simulink model "FMC_TopLevel_Model"  (R2025a)
settings: Solver=VariableStepAuto  StartTime=0.0  StopTime=10.0  RelTol=1e-3
settings Model: Creator=mu22504  LastModifiedBy=Adam

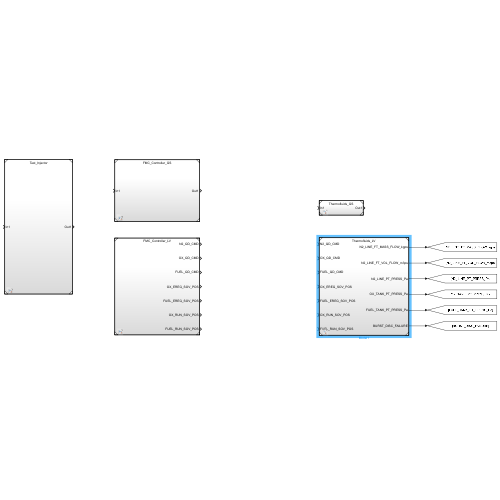
[thumbnail: Simulink's stored preview of the top-level diagram]
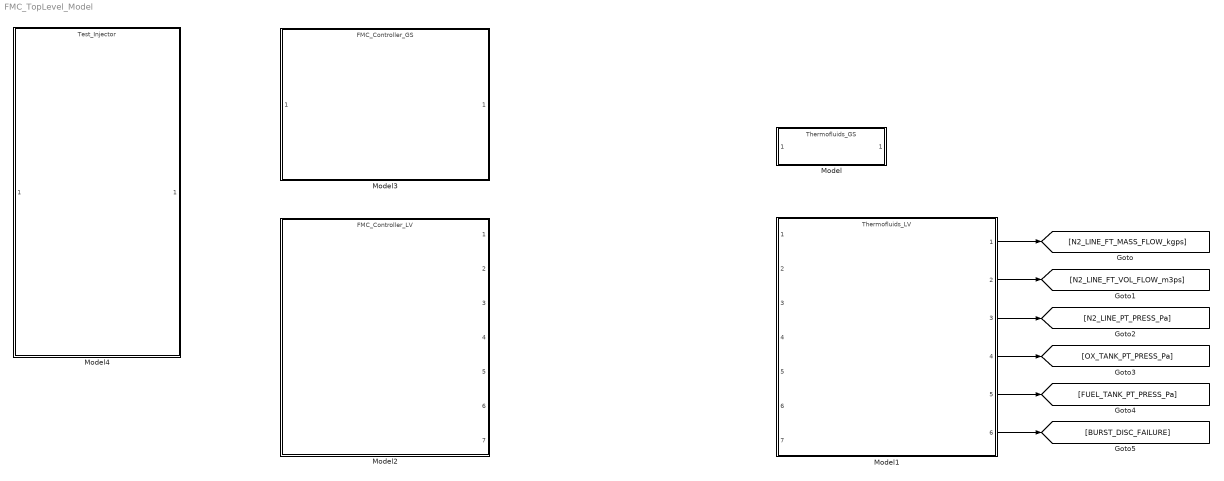
== system FMC_TopLevel_Model ==
  Model : ModelReference  ModelNameDialog=Thermofluids_GS.slx  SimulationMode=Normal  ModelReferenceVersion=1.1
  Model1 : ModelReference  ModelNameDialog=Thermofluids_LV.slx  SimulationMode=Normal  ModelReferenceVersion=1.9
  Model2 : ModelReference  ModelNameDialog=FMC_Controller_LV  SimulationMode=Normal  ModelReferenceVersion=1.2
  Model3 : ModelReference  ModelNameDialog=FMC_Controller_GS  SimulationMode=Normal  ModelReferenceVersion=1.2
  Model4 : ModelReference  ModelNameDialog=Test_Injector.slx  SimulationMode=Normal  ModelReferenceVersion=1.1
  wires:
  Model1/1 -> [N2_LINE_FT_MASS_FLOW_kgps]
  Model1/2 -> [N2_LINE_FT_VOL_FLOW_m3ps]
  Model1/3 -> [N2_LINE_PT_PRESS_Pa]
  Model1/4 -> [OX_TANK_PT_PRESS_Pa]
  Model1/5 -> [FUEL_TANK_PT_PRESS_Pa]
  Model1/6 -> [BURST_DISC_FAILURE]
